simulink model "ImplementingFrictionComp(atSomePoint)"  (R2014a)
settings: Solver=ode1  StartTime=0.0  StopTime=10  FixedStep=0.005  RelTol=1e-3
libraries: c6xlib x2, fricblocks x1
Description:
  | Real-Time Van der Pol Simulation
  | 
  | This demonstration shows a real-time version of the Simulink(R) Van der Pol
  | simulation demo. This model does not need any external signals, so it does
  | not need any data acquisition hardware or driver. This makes the model ideal
  | for first experiments with Real-Time Windows Target(TM), without need to
  | worry about proper I/O hardware configuration.
  | 
  | How to run this demo:
  | 
  |   1. Build the model using Tools -> Real-Time Workshop -> Build Model.
  |   2. Connect to the real-time code using Simulation -> Connect to target.
  |   3. Start the real-time execution using Simulation -> Start real-time code.
settings Model: SimulationMode=external  ExtModeTrigDuration=50000  Creator=Houska  LastModifiedBy=nandi2
settings DataIOCC: SignalLoggingSaveFormat=ModelDataLogs  SignalLoggingName=logsOut
settings OptimizationCC: ExpressionDepthLimit=2147483647  InitFltsAndDblsToZero=on  EfficientMapNaN2IntZero=off
settings DebuggingCC: UnderspecifiedInitializationDetection=Classic  SignalResolutionControl=TryResolveAllWithWarning  SolverPrmCheckMsg=none  FcnCallInpInsideContextMsg=UseLocalSettings  StateNameClashWarn=warning
settings HardwareCC: ProdIntDivRoundTo=Zero  ProdEndianess=LittleEndian  ProdHWDeviceType=32-bit Real-Time Windows Target
settings RTWCC: SystemTargetFile=rtwin.tlc  TemplateMakefile=rtwin.tmf  Description=Real-Time Windows Target  ProcessScript=rtwin_make_rtw_hook
settings RTWinTargetCC: TargetLibSuffix=_rtwin.lib  TargetPreCompLibLocation=C:\MATLABR2014a\toolbox\rtw\targets\rtwin\lib\win64

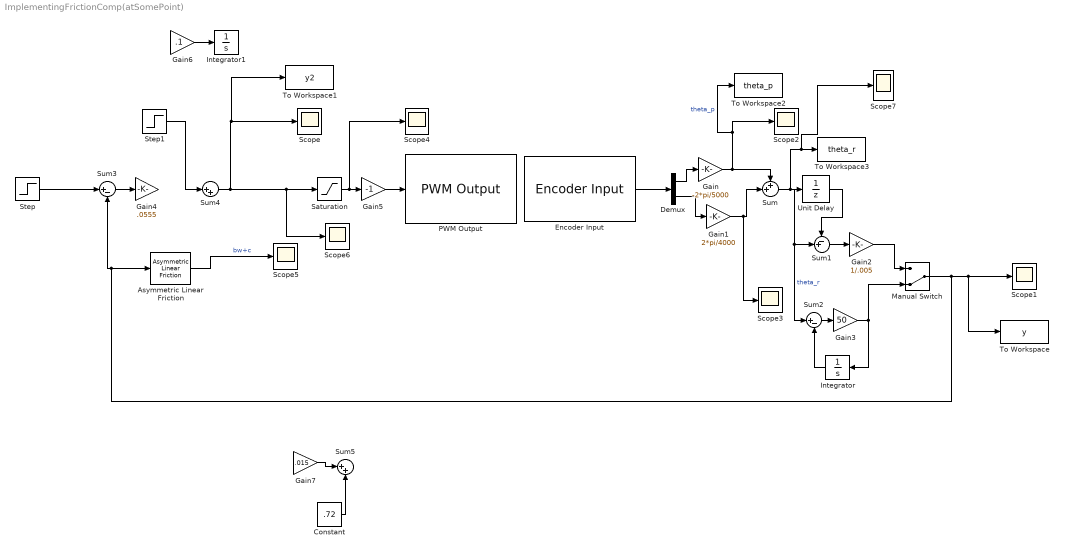
== system ImplementingFrictionComp(atSomePoint) ==
  Asymmetric Linear Friction : fricblocks/Asymmetric  Linear Friction  intercept1=.72  intercept2=-.76  slope1=.015  slope2=.016
  Constant : Constant  Value=.72
  Demux : Demux  Outputs=2
  Encoder Input : c6xlib/Encoder Input  baseAddr=0x378  channels=[0 1]  sampleTime=str2num(get_param(bdroot, 'FixedStep'))
  Gain : Gain  Gain=-2*pi/5000
  Gain1 : Gain  Gain=2*pi/4000
  Gain2 : Gain  Gain=1/.005
  Gain3 : Gain  Gain=50
  Gain4 : Gain  Gain=.0555
  Gain5 : Gain  Gain=-1
  Gain6 : Gain  Gain=.1
  Gain7 : Gain  Gain=.015
  Integrator : Integrator
  Integrator1 : Integrator
  Manual Switch : ManualSwitch  CurrentSetting=0
  PWM Output : c6xlib/PWM Output  baseAddr=0x378  channels=0  initialOutputs=0  finalOutputs=0  sampleTime=str2num(get_param(bdroot, 'FixedStep'))
  Saturation : Saturate  UpperLimit=10  LowerLimit=-10
  Scope{,1..7} (8 alike) : Scope
      Scope1 settings: YMin=315.4  YMax=316.35
      Scope2 settings: YMin=-1.75  YMax=1.75  SaveName=ScopeData2
      Scope3 settings: YMin=-15000  YMax=15000  SaveName=ScopeData3
      Scope4 settings: YMin=0.0555  YMax=0.0555  SaveName=ScopeData4
      Scope5 settings: YMin=9.1  YMax=9.5  SaveName=ScopeData5
      Scope6 settings: YMin=14.05  YMax=14.85  SaveName=ScopeData6
      Scope7 settings: YMin=0  YMax=1800  SaveName=ScopeData7
  Step : Step  Time=0  After=5  SampleTime=0
  Step1 : Step  Time=0  After=5  SampleTime=0
  Sum : Sum  Inputs=++|
  Sum1 : Sum  Inputs=-+|
  Sum2 : Sum  Inputs=|+-
  Sum3 : Sum  Inputs=|+-
  Sum4 : Sum  Inputs=|++
  Sum5 : Sum  Inputs=|++
  To Workspace : ToWorkspace  VariableName=y  SampleTime=-1
  To Workspace1 : ToWorkspace  VariableName=y2  SampleTime=-1
  To Workspace2 : ToWorkspace  VariableName=theta_p  SampleTime=-1
  To Workspace3 : ToWorkspace  VariableName=theta_r  SampleTime=-1
  Unit Delay : UnitDelay  SampleTime=-1
  wires:
  Demux/2 -> Gain1/1
  Demux/1 -> Gain/1
  Encoder Input/1 -> Demux/1
  Gain/1 -> To Workspace2/1, Scope2/1, Sum/1  "theta_p"
  Gain1/1 -> Scope3/1, Sum/2
  Sum/1 -> Scope7/1, To Workspace3/1, Sum2/1, Sum1/2, Unit Delay/1  "theta_r"
  Unit Delay/1 -> Sum1/1
  Sum1/1 -> Gain2/1
  Gain2/1 -> Manual Switch/1
  Integrator/1 -> Sum2/2
  Sum2/1 -> Gain3/1
  Gain3/1 -> Integrator/1, Manual Switch/2
  Step/1 -> Sum3/1
  Manual Switch/1 -> To Workspace/1, Scope1/1, Asymmetric Linear Friction/1, Sum3/2
  Saturation/1 -> Scope4/1, Gain5/1
  Sum3/1 -> Gain4/1
  Sum4/1 -> Scope6/1, Saturation/1, To Workspace1/1, Scope/1
  Gain6/1 -> Integrator1/1
  Gain7/1 -> Sum5/1
  Constant/1 -> Sum5/2
  Asymmetric Linear Friction/1 -> Scope5/1  "bw+c"
  Gain5/1 -> PWM Output/1
  Step1/1 -> Sum4/1
